simulink model "estanque_pid"  (R2025b)
settings: Solver=ode45  StartTime=0.0  StopTime=300  MaxStep=0.1  RelTol=1e-6
values from neighbouring files (symbols this model uses):
  Qin_max = 3e-4    (= 0.0003)    [exportar_csv.m]
undefined symbols (not defined in the file or in its folder): A, beta, h_max, Kd, Ki, Kp, SP_value, theta
libraries: slpidlib x1, simulink x1
settings Model: Creator=benja  LastModifiedBy=benja
settings DataIOCC: SaveFormat=Array

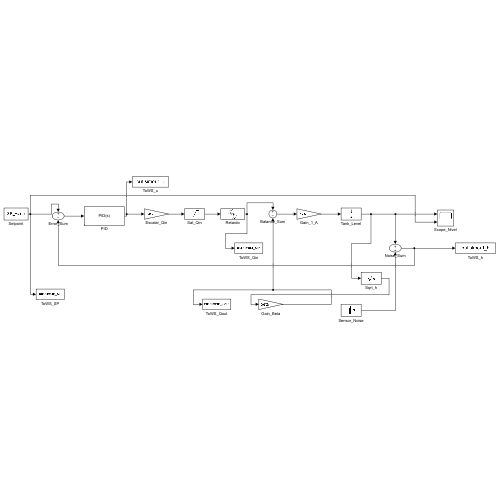
[thumbnail: Simulink's stored preview of the top-level diagram]
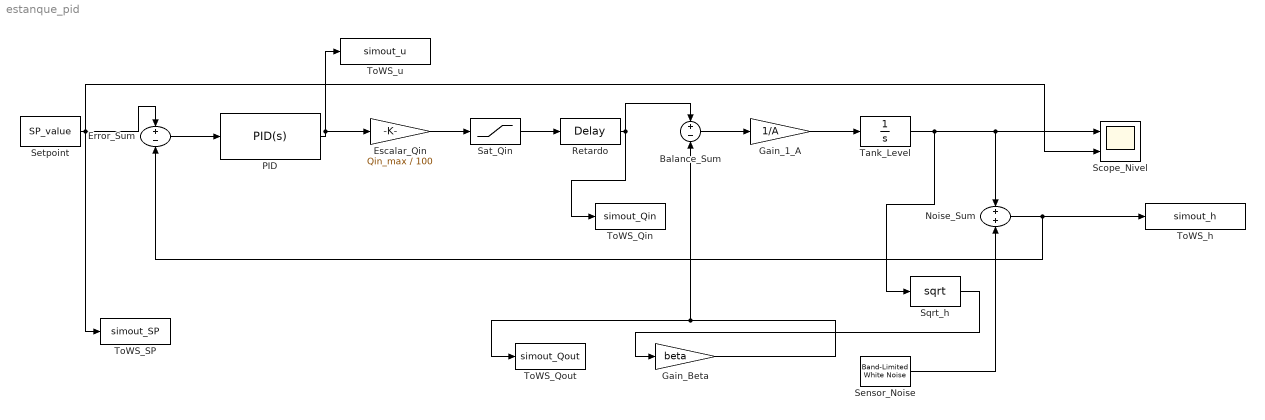
== system estanque_pid ==
  Balance_Sum : Sum  Inputs=+-
  Error_Sum : Sum  Inputs=+-
  Escalar_Qin : Gain  Gain=Qin_max / 100
  Gain_1_A : Gain  Gain=1/A
  Gain_Beta : Gain  Gain=beta
  Noise_Sum : Sum
  PID : slpidlib/PID Controller  Controller=PID  Form=Parallel  TimeDomain=Continuous-time  UseExternalTs=off  SampleTime=-1  IntegratorMethod=Forward Euler  FilterMethod=Forward Euler  ControllerParametersSource=internal  P=Kp  I=Ki  UseKiTs=off  D=Kd  UseExternalDerivativeSource=off  N=100  UseFilter=on  TunerSelectOption=Transfer Function Based (PID Tuner App)  InitialConditionSource=internal  InitialConditionForIntegrator=0  InitialConditionForFilter=0  DifferentiatorICPrevScaledInput=0  ExternalReset=none  TrackingMode=off  Kt=1  LimitOutput=off  SatLimitsSource=internal  UpperSaturationLimit=100  LowerSaturationLimit=0  LinearizeAsGain=on  AntiWindupMode=back-calculation  Kb=1  LimitIntegrator=off  UpperIntegratorSaturationLimit=inf  LowerIntegratorSaturationLimit=-inf  POutMin=[]  POutMax=[]  IOutMin=[]  IOutMax=[]  DOutMin=[]  DOutMax=[]  NOutMin=[]  NOutMax=[]  SumOutMin=[]  SumOutMax=[]  SaturationOutMin=[]  SaturationOutMax=[]  PParamMin=[]  PParamMax=[]  IParamMin=[]  IParamMax=[]  DParamMin=[]  DParamMax=[]  NParamMin=[]  NParamMax=[]  KbParamMin=[]  KbParamMax=[]  KtParamMin=[]  KtParamMax=[]  KbOutMin=[]  KbOutMax=[]  KtOutMin=[]  KtOutMax=[]  IntegratorOutMin=[]  IntegratorOutMax=[]  FilterOutMin=[]  FilterOutMax=[]  SumI1OutMin=[]  SumI1OutMax=[]  SumI2OutMin=[]  SumI2OutMax=[]  SumI3OutMin=[]  SumI3OutMax=[]  SumI4OutMin=[]  SumI4OutMax=[]  SumDOutMin=[]  SumDOutMax=[]  DifferentiatorOutMin=[]  DifferentiatorOutMax=[]  FilterDiffOutCoefMin=[]  FilterDiffOutCoefMax=[]  ReciprocalOutMin=[]  ReciprocalOutMax=[]  SumDenOutMin=[]  SumDenOutMax=[]  SumNumOutMin=[]  SumNumOutMax=[]  DivideOutMin=[]  DivideOutMax=[]  UdiffTsProdOutMin=[]  UdiffTsProdOutMax=[]  NTsProdOutMin=[]  NTsProdOutMax=[]  UintegralTsProdOutMin=[]  UintegralTsProdOutMax=[]  UngainTsProdOutMin=[]  UngainTsProdOutMax=[]  ClampingZeroOutDataTypeStr=Inherit: Inherit via back propagation  ClampingZeroOutMin=[]  ClampingZeroOutMax=[]  FilterDenConstantOutDataTypeStr=Inherit: Inherit via back propagation  FilterDenConstantOutMin=[]  FilterDenConstantOutMax=[]  PCopyOutDataTypeStr=Inherit: Inherit via back propagation  PCopyOutMin=[]  PCopyOutMax=[]  NCopyOutDataTypeStr=Inherit: Inherit via back propagation  NCopyOutMin=[]  NCopyOutMax=[]  IntegratorContinuousStateAttributes=''  IntegratorStateMustResolveToSignalObject=off  IntegratorRTWStateStorageClass=Auto  FilterContinuousStateAttributes=''  FilterStateMustResolveToSignalObject=off  FilterRTWStateStorageClass=Auto  ParallelPVariant=InternalParameters  IdealPVariant=Disabled  IVariant=InternalParameters  DVariant=InternalParameters  IntegratorVariant=Continuous  SatVariant=Disabled  AWVariant=Passthrough  PCopyVariant=Disabled  TRVariant=Disabled  FdbkBlocksVariant=Forward  IdealPFdbkVariant=Disabled  SatFdbkVariant=Disabled  DerivativeFilterVariant=ContFilter  NVariant=InternalParameters  NCopyVariant=Disabled  FilterICVariant=InternalICsFilter  IntegratorICVariant=InternalICs  ExternalResetVariant=Disabled  TRSumVariant=Passthrough  SumFdbkVariant=Disabled  SumVariant=Sum_PID  TsampFilterVariant=InternalTs  TsampNgainVariant=Passthrough  TsampIntegralVariant=Disabled_SignalSpec  ExternalSaturationOutDataTypeStr=Inherit: Same as second input  DerivativeSourceVariant=ErrorSignal  PreIntVariant=InternalPreInt
  Retardo : TransportDelay  DelayTime=theta
  Sat_Qin : Saturate  UpperLimit=Qin_max  LowerLimit=0
  Scope_Nivel : Scope  NumInputPorts=2
  Sensor_Noise : simulink/Sources/Band-Limited White Noise  Cov=2.5e-7  Ts=0.1  seed=[23341]
  Setpoint : Constant  Value=SP_value
  Sqrt_h : Math  Operator=sqrt
  Tank_Level : Integrator  UpperSaturationLimit=h_max  LowerSaturationLimit=0
  ToWS_Qin : ToWorkspace  VariableName=simout_Qin  SaveFormat=Timeseries  SampleTime=-1
  ToWS_Qout : ToWorkspace  VariableName=simout_Qout  SaveFormat=Timeseries  SampleTime=-1
  ToWS_SP : ToWorkspace  VariableName=simout_SP  SaveFormat=Timeseries  SampleTime=-1
  ToWS_h : ToWorkspace  VariableName=simout_h  SaveFormat=Timeseries  SampleTime=-1
  ToWS_u : ToWorkspace  VariableName=simout_u  SaveFormat=Timeseries  SampleTime=-1
  wires:
  Setpoint/1 -> Scope_Nivel/2, Error_Sum/1, ToWS_SP/1
  Error_Sum/1 -> PID/1
  PID/1 -> Escalar_Qin/1, ToWS_u/1
  Escalar_Qin/1 -> Sat_Qin/1
  Sat_Qin/1 -> Retardo/1
  Retardo/1 -> Balance_Sum/1, ToWS_Qin/1
  Balance_Sum/1 -> Gain_1_A/1
  Gain_1_A/1 -> Tank_Level/1
  Tank_Level/1 -> Scope_Nivel/1, Noise_Sum/1, Sqrt_h/1
  Sensor_Noise/1 -> Noise_Sum/2
  Noise_Sum/1 -> ToWS_h/1, Error_Sum/2
  Sqrt_h/1 -> Gain_Beta/1
  Gain_Beta/1 -> Balance_Sum/2, ToWS_Qout/1
